simulink model "Assignment_4"  (R2020b)
settings: Solver=VariableStepAuto  StartTime=0.0  StopTime=0.2  RelTol=1e-3
values from neighbouring files (symbols this model uses):
  b = 3.5077E-6    [Dict_Assignment_4.sldd]
  J = 3.2284E-6    [Dict_Assignment_4.sldd]
  K = 0.0274    [Dict_Assignment_4.sldd]
  L = 2.75E-6    [Dict_Assignment_4.sldd]
  R = 4.0    [Dict_Assignment_4.sldd]
settings Model: DataDictionary=Dict_Assignment_4.sldd  Creator=Shantam Garg  LastModifiedBy=Shantam Garg

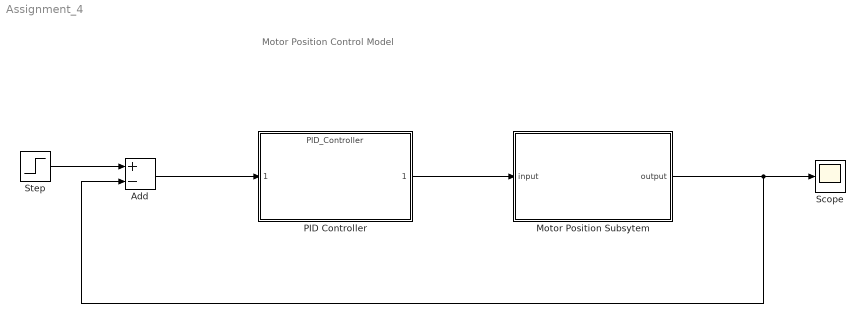
== system Assignment_4 ==
  note: Motor Position Control Model
  Add : Sum  Inputs=+-
  Motor Position Subsytem : Subsystem
  PID Controller : ModelReference  ModelNameDialog=PID_Controller  SimulationMode=Normal  ModelReferenceVersion=1.5
  Scope : Scope
  Step : Step  Time=0  SampleTime=0
  wires:
  Motor Position Subsytem/1(output) -> Add/2, Scope/1
  Step/1 -> Add/1
  Add/1 -> PID Controller/1
  PID Controller/1 -> Motor Position Subsytem/1(input)

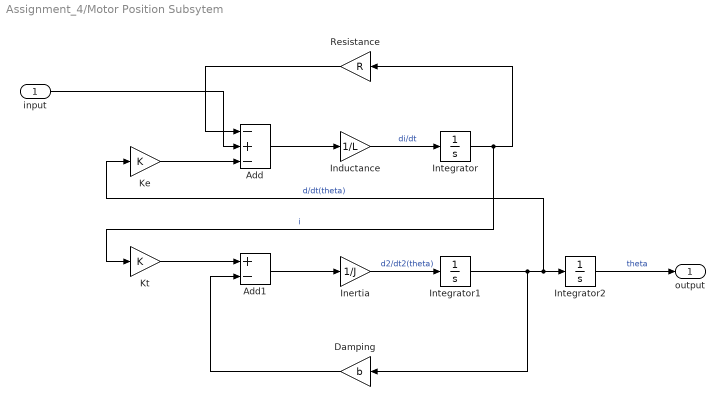
== system Assignment_4/Motor Position Subsytem ==
  input : Inport
  Add : Sum  Inputs=-+-
  Add1 : Sum  Inputs=+-
  Damping : Gain  Gain=b
  Inductance : Gain  Gain=1/L
  Inertia : Gain  Gain=1/J
  Integrator : Integrator
  Integrator1 : Integrator
  Integrator2 : Integrator
  Ke : Gain  Gain=K
  Kt : Gain  Gain=K
  Resistance : Gain  Gain=R
  output : Outport
  wires:
  Add/1 -> Inductance/1
  Integrator/1 -> Resistance/1, Kt/1  "i"
  Add1/1 -> Inertia/1
  Inductance/1 -> Integrator/1  "di/dt"
  Inertia/1 -> Integrator1/1  "d2/dt2(theta)"
  Kt/1 -> Add1/1
  Ke/1 -> Add/3
  Integrator1/1 -> Ke/1, Integrator2/1, Damping/1  "d/dt(theta)"
  Resistance/1 -> Add/1
  input/1 -> Add/2
  Damping/1 -> Add1/2
  Integrator2/1 -> output/1  "theta"
